simulink model "simTrabalho_CDU_sem_Desacoplador"  (R2018b)
settings: Solver=VariableStepAuto  StartTime=0.0  StopTime=tsim  MaxStep=1/10  RelTol=1e-3  EnableMultiTasking=on
values from neighbouring files (symbols this model uses):
  D = minreal(D)    [main.m]
  Dn = D    [main.m]
  G = G(iy,iu)    [main.m]
  u0 = u0(iu)    [main.m]
  umax = umax(iu)    [main.m]
  umin = umin(iu)    [main.m]
  y0 = y0(iy)    [main.m]
  ymax = ymax(iy)    [main.m]
  ymin = ymin(iy)    [main.m]
undefined symbols (not defined in the file or in its folder): Tdio
libraries: cstextras x36
settings Model: Creator=treezao  LastModifiedBy=Aluno
settings OptimizationCC: LifeSpan=inf
settings DebuggingCC: LibraryContextMissingDiagnostic=none  SFUnexpectedBacktrackingDiag=warning  SFNoUnconditionalDefaultTransitionDiag=warning  SFExecutionAtInitializationDiag=none
settings SFSimCC: SimUseLocalCustomCode=off
settings RTWCC: RTWUseLocalCustomCode=off
settings CodeAppCC: StateflowObjectComments=on
settings GRTTargetCC: TargetLangStandard=C89/C90 (ANSI)  GeneratePreprocessorConditionals=Disable all
settings ConfigComp: CovMetricSettings=dw  CovHtmlReporting=on  CovSaveCumulativeToWorkspaceVar=on  CovSaveSingleToWorkspaceVar=on  CovExternalEMLEnable=off

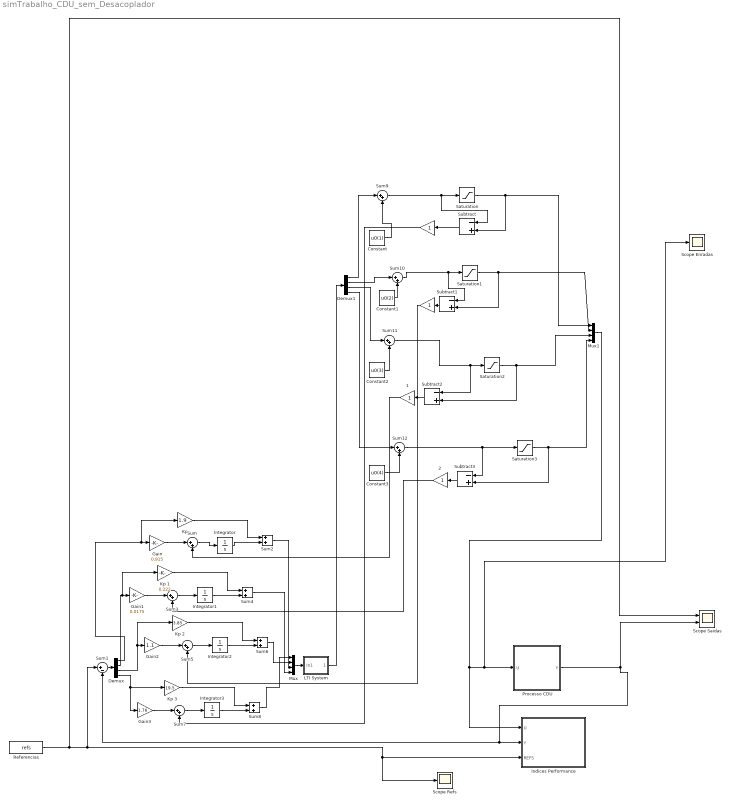
== system simTrabalho_CDU_sem_Desacoplador ==
   {,,1..2} (4 alike) : Gain
  Constant : Constant  Value=u0(1)
  Constant1 : Constant  Value=u0(2)
  Constant2 : Constant  Value=u0(3)
  Constant3 : Constant  Value=u0(4)
  Demux : Demux
  Demux1 : Demux
  Gain : Gain  Gain=0.915
  Gain1 : Gain  Gain=0.0175
  Gain2 : Gain  Gain=1.1
  Gain3 : Gain  Gain=1.76
  Indices Performance : Subsystem
  Integrator{,1..3} (4 alike) : Integrator
  "Kp " : Gain  Gain=1.9
  Kp 1 : Gain  Gain=0.222
  Kp 2 : Gain  Gain=3.85
  Kp 3 : Gain  Gain=19.5
  LTI System : Subsystem  AncestorBlock=cstblocks/LTI System  BlockChoice=CSS  mask(LTI Block){sys=Dn, IC=[]}
      mask prompts: sys "Control:simulink:LTIMaskLabel1"; IC "Control:simulink:LTIMaskLabel2"
      mask help: Control:simulink:LTIMaskDescription
      mask init:
      | try
      |    % read data to initialize mask variables
      |    [D,Ts,Tdi,Tdo,Tdio,x0,sysname]=...
      |       ltimask('Initialize',gcb,sys,IC);
      |    % update contents
      |    model = bdroot;
      |    df = get_param(model,'dirty');
      |    ltimask('UpdateDiagram',gcb,D,Ts,Tdio);
      |    try      
      |       % Attempt to modify locked library -> error
      |       % Makes block show ??? when loading CSTBLOCKS
      |       % for the first time
      |       set_param(model,'dirty',df)
      |    end
      | catch ME
      |    sys = [];  IC = [];   sysname = '???';
      |    throw(ME)
      | end
      mask Help: eval('ctrlguihelp(''ltisystemblock'');')
      mask Callback sys: ltimask('MaskLTICallback',gcb);
      mask Display: disp(sysname)
  Mux : Mux
  Mux1 : Mux
  Processo CDU : Subsystem
  Referencias : FromWorkspace  VariableName=refs  SampleTime=0  Interpolate=off  OutputAfterFinalValue=Holding final value
  Saturation : Saturate  UpperLimit=umax(1)  LowerLimit=umin(1)  LinearizeAsGain=off
  Saturation1 : Saturate  UpperLimit=umax(2)  LowerLimit=umin(2)  LinearizeAsGain=off
  Saturation2 : Saturate  UpperLimit=umax(3)  LowerLimit=umin(3)  LinearizeAsGain=off
  Saturation3 : Saturate  UpperLimit=umax(4)  LowerLimit=umin(4)  LinearizeAsGain=off
  Scope Enradas : Scope
  Scope Refs : Scope
  Scope Saidas : Scope  NumInputPorts=2
  Subtract{,1..3} (4 alike) : Sum  Inputs=-+
  Sum{,3,5,7,9..12} (8 alike) : Sum  Inputs=|++
  Sum1 : Sum  Inputs=|+-
  Sum{2,4,6,8} (4 alike) : Sum
  wires:
  Referencias/1 -> Scope Refs/1, Indices Performance/3(REFS), Sum1/1, Scope Saidas/1
  Demux/1 -> "Kp "/1, Gain/1
  Demux/2 -> Kp 1/1, Gain1/1
  Demux/3 -> Kp 2/1, Gain2/1
  Demux/4 -> Gain3/1, Kp 3/1
  Sum2/1 -> Mux/3
  Sum4/1 -> Mux/4
  Sum8/1 -> Mux/1
  Processo CDU/1(Y) -> Indices Performance/2(Y), Sum1/2, Scope Saidas/2
  Sum1/1 -> Demux/1
  Mux/1 -> LTI System/1(In1)
  Sum/1 -> Integrator/1
  Integrator/1 -> Sum2/2
  Gain/1 -> Sum/1
  "Kp "/1 -> Sum2/1
  Sum3/1 -> Integrator1/1
  Integrator1/1 -> Sum4/2
  Gain1/1 -> Sum3/1
  Kp 1/1 -> Sum4/1
  Sum5/1 -> Integrator2/1
  Integrator2/1 -> Sum6/2
  Gain2/1 -> Sum5/1
  Kp 2/1 -> Sum6/1
  Sum6/1 -> Mux/2
  Sum7/1 -> Integrator3/1
  Integrator3/1 -> Sum8/2
  Gain3/1 -> Sum7/1
  Kp 3/1 -> Sum8/1
  Subtract/1 -> " "/1
  Saturation/1 -> Subtract/2, Mux1/1
  Subtract1/1 -> " "/1
  Subtract2/1 -> " 1"/1
  Saturation1/1 -> Subtract1/2, Mux1/2
  Saturation2/1 -> Subtract2/2, Mux1/3
  Subtract3/1 -> " 2"/1
  Saturation3/1 -> Subtract3/2, Mux1/4
  Mux1/1 -> Indices Performance/1(U), Processo CDU/1(U), Scope Enradas/1
  LTI System/1(Out1) -> Demux1/1
  Sum9/1 -> Subtract/1, Saturation/1
  Demux1/1 -> Sum9/1
  Demux1/2 -> Sum10/1
  Sum10/1 -> Subtract1/1, Saturation1/1
  Demux1/3 -> Sum11/1
  Sum11/1 -> Subtract2/1, Saturation2/1
  Demux1/4 -> Sum12/1
  Sum12/1 -> Subtract3/1, Saturation3/1
  Constant/1 -> Sum9/2
  Constant1/1 -> Sum10/2
  Constant2/1 -> Sum11/2
  Constant3/1 -> Sum12/2
  " "/1 -> Sum5/2
  " "/1 -> Sum7/2
  " 1"/1 -> Sum/2
  " 2"/1 -> Sum3/2

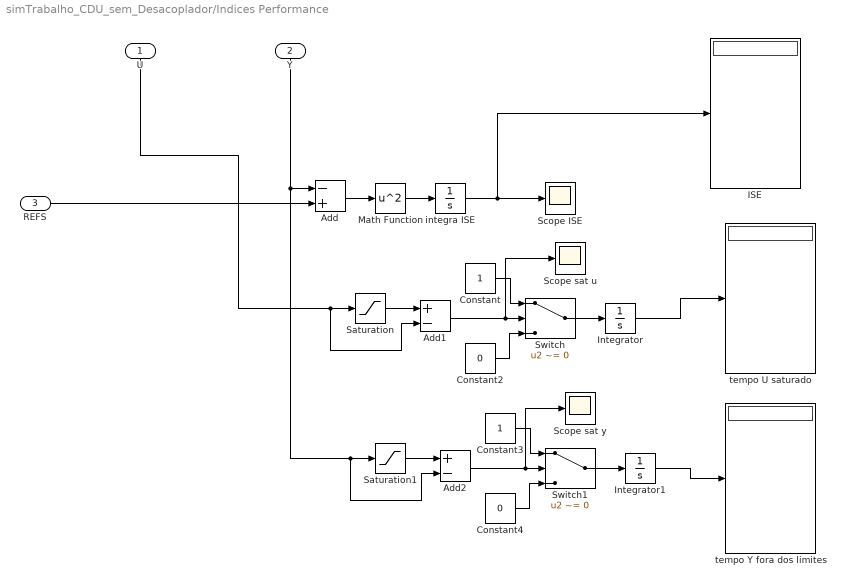
== system simTrabalho_CDU_sem_Desacoplador/Indices Performance ==
  U : Inport
  Y : Inport  Port=2
  REFS : Inport  Port=3
  Add : Sum  Inputs=-+
  Add1 : Sum  Inputs=+-
  Add2 : Sum  Inputs=+-
  Constant : Constant
  Constant2 : Constant  Value=0
  Constant3 : Constant
  Constant4 : Constant  Value=0
  ISE : Display
  Integrator : Integrator
  Integrator1 : Integrator
  Math Function : Math  Operator=square  SaturateOnIntegerOverflow=on
  Saturation : Saturate  UpperLimit=umax  LowerLimit=umin
  Saturation1 : Saturate  UpperLimit=ymax  LowerLimit=ymin
  Scope ISE : Scope
  Scope sat u : Scope
  Scope sat y : Scope
  Switch : Switch  Criteria=u2 ~= 0
  Switch1 : Switch  Criteria=u2 ~= 0
  integra ISE : Integrator
  tempo U saturado : Display
  tempo Y fora dos limites : Display
  wires:
  REFS/1 -> Add/2
  Y/1 -> Add2/2, Saturation1/1, Add/1
  U/1 -> Add1/2, Saturation/1
  Add2/1 -> Scope sat y/1, Switch1/2
  Constant3/1 -> Switch1/1
  Integrator1/1 -> tempo Y fora dos limites/1
  Constant4/1 -> Switch1/3
  Switch1/1 -> Integrator1/1
  Saturation1/1 -> Add2/1
  Saturation/1 -> Add1/1
  Constant2/1 -> Switch/3
  integra ISE/1 -> ISE/1, Scope ISE/1
  Constant/1 -> Switch/1
  Integrator/1 -> tempo U saturado/1
  Switch/1 -> Integrator/1
  Add1/1 -> Switch/2, Scope sat u/1
  Math Function/1 -> integra ISE/1
  Add/1 -> Math Function/1

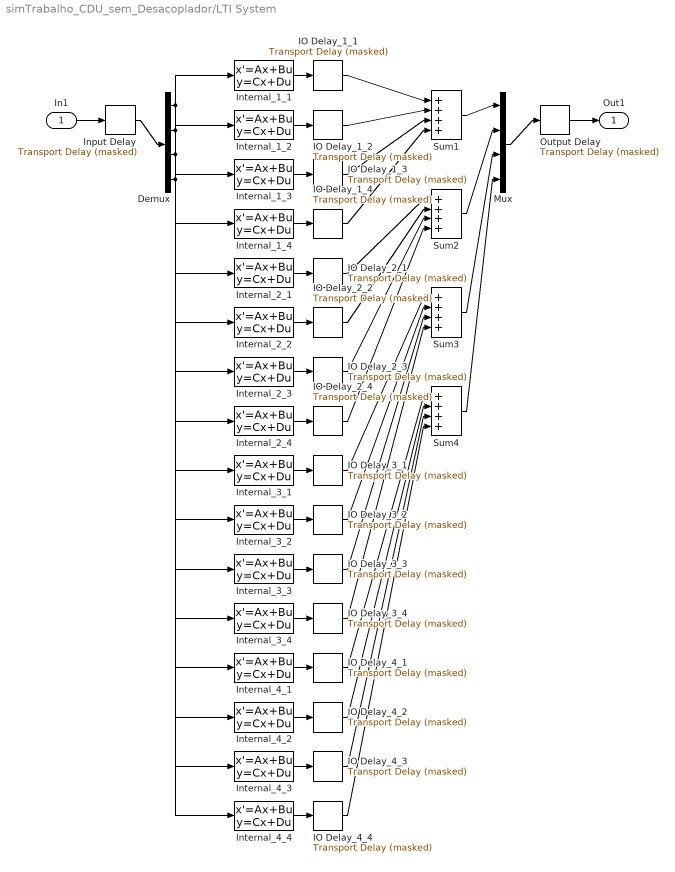
== system simTrabalho_CDU_sem_Desacoplador/LTI System ==
  In1 : Inport
  Demux : Demux
  IO Delay_1_1 : cstextras/Transport Delay (masked)  Td=Tdio(1,1)  u0=0  bufsize=1024
      settings: SourceProductName=Control System Toolbox  SourceProductBaseCode=CT
  IO Delay_1_2 : cstextras/Transport Delay (masked)  Td=Tdio(1,2)  u0=0  bufsize=1024
      settings: SourceProductName=Control System Toolbox  SourceProductBaseCode=CT
  IO Delay_1_3 : cstextras/Transport Delay (masked)  Td=Tdio(1,3)  u0=0  bufsize=1024
      settings: SourceProductName=Control System Toolbox  SourceProductBaseCode=CT
  IO Delay_1_4 : cstextras/Transport Delay (masked)  Td=Tdio(1,4)  u0=0  bufsize=1024
      settings: SourceProductName=Control System Toolbox  SourceProductBaseCode=CT
  IO Delay_2_1 : cstextras/Transport Delay (masked)  Td=Tdio(2,1)  u0=0  bufsize=1024
      settings: SourceProductName=Control System Toolbox  SourceProductBaseCode=CT
  IO Delay_2_2 : cstextras/Transport Delay (masked)  Td=Tdio(2,2)  u0=0  bufsize=1024
      settings: SourceProductName=Control System Toolbox  SourceProductBaseCode=CT
  IO Delay_2_3 : cstextras/Transport Delay (masked)  Td=Tdio(2,3)  u0=0  bufsize=1024
      settings: SourceProductName=Control System Toolbox  SourceProductBaseCode=CT
  IO Delay_2_4 : cstextras/Transport Delay (masked)  Td=Tdio(2,4)  u0=0  bufsize=1024
      settings: SourceProductName=Control System Toolbox  SourceProductBaseCode=CT
  IO Delay_3_1 : cstextras/Transport Delay (masked)  Td=Tdio(3,1)  u0=0  bufsize=1024
      settings: SourceProductName=Control System Toolbox  SourceProductBaseCode=CT
  IO Delay_3_2 : cstextras/Transport Delay (masked)  Td=Tdio(3,2)  u0=0  bufsize=1024
      settings: SourceProductName=Control System Toolbox  SourceProductBaseCode=CT
  IO Delay_3_3 : cstextras/Transport Delay (masked)  Td=Tdio(3,3)  u0=0  bufsize=1024
      settings: SourceProductName=Control System Toolbox  SourceProductBaseCode=CT
  IO Delay_3_4 : cstextras/Transport Delay (masked)  Td=Tdio(3,4)  u0=0  bufsize=1024
      settings: SourceProductName=Control System Toolbox  SourceProductBaseCode=CT
  IO Delay_4_1 : cstextras/Transport Delay (masked)  Td=Tdio(4,1)  u0=0  bufsize=1024
      settings: SourceProductName=Control System Toolbox  SourceProductBaseCode=CT
  IO Delay_4_2 : cstextras/Transport Delay (masked)  Td=Tdio(4,2)  u0=0  bufsize=1024
      settings: SourceProductName=Control System Toolbox  SourceProductBaseCode=CT
  IO Delay_4_3 : cstextras/Transport Delay (masked)  Td=Tdio(4,3)  u0=0  bufsize=1024
      settings: SourceProductName=Control System Toolbox  SourceProductBaseCode=CT
  IO Delay_4_4 : cstextras/Transport Delay (masked)  Td=Tdio(4,4)  u0=0  bufsize=1024
      settings: SourceProductName=Control System Toolbox  SourceProductBaseCode=CT
  Input Delay : cstextras/Transport Delay (masked)  Td=Tdi  u0=0  bufsize=1024
      settings: SourceProductName=Control System Toolbox  SourceProductBaseCode=CT
  Internal_1_1 : StateSpace  A=D(1,1).a  B=D(1,1).b  C=D(1,1).c  D=D(1,1).d
  Internal_1_2 : StateSpace  A=D(1,2).a  B=D(1,2).b  C=D(1,2).c  D=D(1,2).d
  Internal_1_3 : StateSpace  A=D(1,3).a  B=D(1,3).b  C=D(1,3).c  D=D(1,3).d
  Internal_1_4 : StateSpace  A=D(1,4).a  B=D(1,4).b  C=D(1,4).c  D=D(1,4).d
  Internal_2_1 : StateSpace  A=D(2,1).a  B=D(2,1).b  C=D(2,1).c  D=D(2,1).d
  Internal_2_2 : StateSpace  A=D(2,2).a  B=D(2,2).b  C=D(2,2).c  D=D(2,2).d
  Internal_2_3 : StateSpace  A=D(2,3).a  B=D(2,3).b  C=D(2,3).c  D=D(2,3).d
  Internal_2_4 : StateSpace  A=D(2,4).a  B=D(2,4).b  C=D(2,4).c  D=D(2,4).d
  Internal_3_1 : StateSpace  A=D(3,1).a  B=D(3,1).b  C=D(3,1).c  D=D(3,1).d
  Internal_3_2 : StateSpace  A=D(3,2).a  B=D(3,2).b  C=D(3,2).c  D=D(3,2).d
  Internal_3_3 : StateSpace  A=D(3,3).a  B=D(3,3).b  C=D(3,3).c  D=D(3,3).d
  Internal_3_4 : StateSpace  A=D(3,4).a  B=D(3,4).b  C=D(3,4).c  D=D(3,4).d
  Internal_4_1 : StateSpace  A=D(4,1).a  B=D(4,1).b  C=D(4,1).c  D=D(4,1).d
  Internal_4_2 : StateSpace  A=D(4,2).a  B=D(4,2).b  C=D(4,2).c  D=D(4,2).d
  Internal_4_3 : StateSpace  A=D(4,3).a  B=D(4,3).b  C=D(4,3).c  D=D(4,3).d
  Internal_4_4 : StateSpace  A=D(4,4).a  B=D(4,4).b  C=D(4,4).c  D=D(4,4).d
  Mux : Mux
  Output Delay : cstextras/Transport Delay (masked)  Td=Tdo  u0=0  bufsize=1024
      settings: SourceProductName=Control System Toolbox  SourceProductBaseCode=CT
  Sum{1..4} (4 alike) : Sum  Inputs=++++  SaturateOnIntegerOverflow=on  InputSameDT=on  OutDataTypeStr=Inherit: Same as first input
  Out1 : Outport  InitialOutput=0
  wires:
  In1/1 -> Input Delay/1
  Output Delay/1 -> Out1/1
  Input Delay/1 -> Demux/1
  Mux/1 -> Output Delay/1
  Sum1/1 -> Mux/1
  Sum2/1 -> Mux/2
  Sum3/1 -> Mux/3
  Sum4/1 -> Mux/4
  Demux/1 -> Internal_1_1/1, Internal_2_1/1, Internal_3_1/1, Internal_4_1/1
  Internal_1_1/1 -> IO Delay_1_1/1
  IO Delay_1_1/1 -> Sum1/1
  Demux/2 -> Internal_1_2/1, Internal_2_2/1, Internal_3_2/1, Internal_4_2/1
  Internal_1_2/1 -> IO Delay_1_2/1
  IO Delay_1_2/1 -> Sum1/2
  Demux/3 -> Internal_1_3/1, Internal_2_3/1, Internal_3_3/1, Internal_4_3/1
  Internal_1_3/1 -> IO Delay_1_3/1
  IO Delay_1_3/1 -> Sum1/3
  Demux/4 -> Internal_1_4/1, Internal_2_4/1, Internal_3_4/1, Internal_4_4/1
  Internal_1_4/1 -> IO Delay_1_4/1
  IO Delay_1_4/1 -> Sum1/4
  Internal_2_1/1 -> IO Delay_2_1/1
  IO Delay_2_1/1 -> Sum2/1
  Internal_2_2/1 -> IO Delay_2_2/1
  IO Delay_2_2/1 -> Sum2/2
  Internal_2_3/1 -> IO Delay_2_3/1
  IO Delay_2_3/1 -> Sum2/3
  Internal_2_4/1 -> IO Delay_2_4/1
  IO Delay_2_4/1 -> Sum2/4
  Internal_3_1/1 -> IO Delay_3_1/1
  IO Delay_3_1/1 -> Sum3/1
  Internal_3_2/1 -> IO Delay_3_2/1
  IO Delay_3_2/1 -> Sum3/2
  Internal_3_3/1 -> IO Delay_3_3/1
  IO Delay_3_3/1 -> Sum3/3
  Internal_3_4/1 -> IO Delay_3_4/1
  IO Delay_3_4/1 -> Sum3/4
  Internal_4_1/1 -> IO Delay_4_1/1
  IO Delay_4_1/1 -> Sum4/1
  Internal_4_2/1 -> IO Delay_4_2/1
  IO Delay_4_2/1 -> Sum4/2
  Internal_4_3/1 -> IO Delay_4_3/1
  IO Delay_4_3/1 -> Sum4/3
  Internal_4_4/1 -> IO Delay_4_4/1
  IO Delay_4_4/1 -> Sum4/4

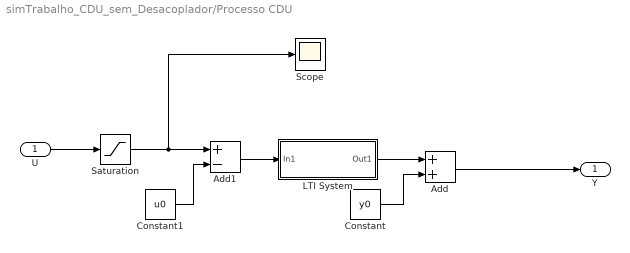
== system simTrabalho_CDU_sem_Desacoplador/Processo CDU ==
  U : Inport
  Add : Sum
  Add1 : Sum  Inputs=+-
  Constant : Constant  Value=y0
  Constant1 : Constant  Value=u0
  LTI System : Subsystem  AncestorBlock=cstblocks/LTI System  BlockChoice=CSS  mask(LTI Block){sys=G, IC=[]}
      mask prompts: sys "Control:simulink:LTIMaskLabel1"; IC "Control:simulink:LTIMaskLabel2"
      mask help: Control:simulink:LTIMaskDescription
      mask init: same as simTrabalho_CDU_sem_Desacoplador/LTI System
      mask Help: eval('ctrlguihelp(''ltisystemblock'');')
      mask Callback sys: ltimask('MaskLTICallback',gcb);
      mask Display: disp(sysname)
  Saturation : Saturate  UpperLimit=umax  LowerLimit=umin
  Scope : Scope
  Y : Outport
  wires:
  LTI System/1(Out1) -> Add/1
  U/1 -> Saturation/1
  Add1/1 -> LTI System/1(In1)
  Constant/1 -> Add/2
  Add/1 -> Y/1
  Constant1/1 -> Add1/2
  Saturation/1 -> Scope/1, Add1/1

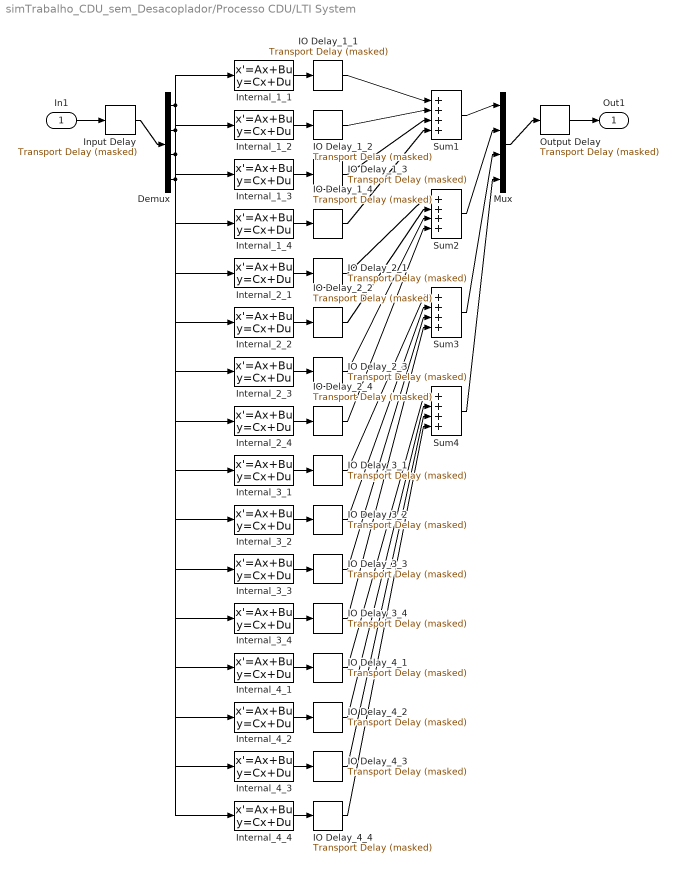
== system simTrabalho_CDU_sem_Desacoplador/Processo CDU/LTI System ==
  In1 : Inport
  Demux : Demux
  IO Delay_1_1 : cstextras/Transport Delay (masked)  Td=Tdio(1,1)  u0=0  bufsize=1024
      settings: SourceProductName=Control System Toolbox  SourceProductBaseCode=CT
  IO Delay_1_2 : cstextras/Transport Delay (masked)  Td=Tdio(1,2)  u0=0  bufsize=1024
      settings: SourceProductName=Control System Toolbox  SourceProductBaseCode=CT
  IO Delay_1_3 : cstextras/Transport Delay (masked)  Td=Tdio(1,3)  u0=0  bufsize=1024
      settings: SourceProductName=Control System Toolbox  SourceProductBaseCode=CT
  IO Delay_1_4 : cstextras/Transport Delay (masked)  Td=Tdio(1,4)  u0=0  bufsize=1024
      settings: SourceProductName=Control System Toolbox  SourceProductBaseCode=CT
  IO Delay_2_1 : cstextras/Transport Delay (masked)  Td=Tdio(2,1)  u0=0  bufsize=1024
      settings: SourceProductName=Control System Toolbox  SourceProductBaseCode=CT
  IO Delay_2_2 : cstextras/Transport Delay (masked)  Td=Tdio(2,2)  u0=0  bufsize=1024
      settings: SourceProductName=Control System Toolbox  SourceProductBaseCode=CT
  IO Delay_2_3 : cstextras/Transport Delay (masked)  Td=Tdio(2,3)  u0=0  bufsize=1024
      settings: SourceProductName=Control System Toolbox  SourceProductBaseCode=CT
  IO Delay_2_4 : cstextras/Transport Delay (masked)  Td=Tdio(2,4)  u0=0  bufsize=1024
      settings: SourceProductName=Control System Toolbox  SourceProductBaseCode=CT
  IO Delay_3_1 : cstextras/Transport Delay (masked)  Td=Tdio(3,1)  u0=0  bufsize=1024
      settings: SourceProductName=Control System Toolbox  SourceProductBaseCode=CT
  IO Delay_3_2 : cstextras/Transport Delay (masked)  Td=Tdio(3,2)  u0=0  bufsize=1024
      settings: SourceProductName=Control System Toolbox  SourceProductBaseCode=CT
  IO Delay_3_3 : cstextras/Transport Delay (masked)  Td=Tdio(3,3)  u0=0  bufsize=1024
      settings: SourceProductName=Control System Toolbox  SourceProductBaseCode=CT
  IO Delay_3_4 : cstextras/Transport Delay (masked)  Td=Tdio(3,4)  u0=0  bufsize=1024
      settings: SourceProductName=Control System Toolbox  SourceProductBaseCode=CT
  IO Delay_4_1 : cstextras/Transport Delay (masked)  Td=Tdio(4,1)  u0=0  bufsize=1024
      settings: SourceProductName=Control System Toolbox  SourceProductBaseCode=CT
  IO Delay_4_2 : cstextras/Transport Delay (masked)  Td=Tdio(4,2)  u0=0  bufsize=1024
      settings: SourceProductName=Control System Toolbox  SourceProductBaseCode=CT
  IO Delay_4_3 : cstextras/Transport Delay (masked)  Td=Tdio(4,3)  u0=0  bufsize=1024
      settings: SourceProductName=Control System Toolbox  SourceProductBaseCode=CT
  IO Delay_4_4 : cstextras/Transport Delay (masked)  Td=Tdio(4,4)  u0=0  bufsize=1024
      settings: SourceProductName=Control System Toolbox  SourceProductBaseCode=CT
  Input Delay : cstextras/Transport Delay (masked)  Td=Tdi  u0=0  bufsize=1024
      settings: SourceProductName=Control System Toolbox  SourceProductBaseCode=CT
  Internal_1_1 : StateSpace  A=D(1,1).a  B=D(1,1).b  C=D(1,1).c  D=D(1,1).d
  Internal_1_2 : StateSpace  A=D(1,2).a  B=D(1,2).b  C=D(1,2).c  D=D(1,2).d
  Internal_1_3 : StateSpace  A=D(1,3).a  B=D(1,3).b  C=D(1,3).c  D=D(1,3).d
  Internal_1_4 : StateSpace  A=D(1,4).a  B=D(1,4).b  C=D(1,4).c  D=D(1,4).d
  Internal_2_1 : StateSpace  A=D(2,1).a  B=D(2,1).b  C=D(2,1).c  D=D(2,1).d
  Internal_2_2 : StateSpace  A=D(2,2).a  B=D(2,2).b  C=D(2,2).c  D=D(2,2).d
  Internal_2_3 : StateSpace  A=D(2,3).a  B=D(2,3).b  C=D(2,3).c  D=D(2,3).d
  Internal_2_4 : StateSpace  A=D(2,4).a  B=D(2,4).b  C=D(2,4).c  D=D(2,4).d
  Internal_3_1 : StateSpace  A=D(3,1).a  B=D(3,1).b  C=D(3,1).c  D=D(3,1).d
  Internal_3_2 : StateSpace  A=D(3,2).a  B=D(3,2).b  C=D(3,2).c  D=D(3,2).d
  Internal_3_3 : StateSpace  A=D(3,3).a  B=D(3,3).b  C=D(3,3).c  D=D(3,3).d
  Internal_3_4 : StateSpace  A=D(3,4).a  B=D(3,4).b  C=D(3,4).c  D=D(3,4).d
  Internal_4_1 : StateSpace  A=D(4,1).a  B=D(4,1).b  C=D(4,1).c  D=D(4,1).d
  Internal_4_2 : StateSpace  A=D(4,2).a  B=D(4,2).b  C=D(4,2).c  D=D(4,2).d
  Internal_4_3 : StateSpace  A=D(4,3).a  B=D(4,3).b  C=D(4,3).c  D=D(4,3).d
  Internal_4_4 : StateSpace  A=D(4,4).a  B=D(4,4).b  C=D(4,4).c  D=D(4,4).d
  Mux : Mux
  Output Delay : cstextras/Transport Delay (masked)  Td=Tdo  u0=0  bufsize=1024
      settings: SourceProductName=Control System Toolbox  SourceProductBaseCode=CT
  Sum{1..4} (4 alike) : Sum  Inputs=++++  SaturateOnIntegerOverflow=on  InputSameDT=on  OutDataTypeStr=Inherit: Same as first input
  Out1 : Outport  InitialOutput=0
  wires:
  In1/1 -> Input Delay/1
  Output Delay/1 -> Out1/1
  Input Delay/1 -> Demux/1
  Mux/1 -> Output Delay/1
  Sum1/1 -> Mux/1
  Sum2/1 -> Mux/2
  Sum3/1 -> Mux/3
  Sum4/1 -> Mux/4
  Demux/1 -> Internal_1_1/1, Internal_2_1/1, Internal_3_1/1, Internal_4_1/1
  Internal_1_1/1 -> IO Delay_1_1/1
  IO Delay_1_1/1 -> Sum1/1
  Demux/2 -> Internal_1_2/1, Internal_2_2/1, Internal_3_2/1, Internal_4_2/1
  Internal_1_2/1 -> IO Delay_1_2/1
  IO Delay_1_2/1 -> Sum1/2
  Demux/3 -> Internal_1_3/1, Internal_2_3/1, Internal_3_3/1, Internal_4_3/1
  Internal_1_3/1 -> IO Delay_1_3/1
  IO Delay_1_3/1 -> Sum1/3
  Demux/4 -> Internal_1_4/1, Internal_2_4/1, Internal_3_4/1, Internal_4_4/1
  Internal_1_4/1 -> IO Delay_1_4/1
  IO Delay_1_4/1 -> Sum1/4
  Internal_2_1/1 -> IO Delay_2_1/1
  IO Delay_2_1/1 -> Sum2/1
  Internal_2_2/1 -> IO Delay_2_2/1
  IO Delay_2_2/1 -> Sum2/2
  Internal_2_3/1 -> IO Delay_2_3/1
  IO Delay_2_3/1 -> Sum2/3
  Internal_2_4/1 -> IO Delay_2_4/1
  IO Delay_2_4/1 -> Sum2/4
  Internal_3_1/1 -> IO Delay_3_1/1
  IO Delay_3_1/1 -> Sum3/1
  Internal_3_2/1 -> IO Delay_3_2/1
  IO Delay_3_2/1 -> Sum3/2
  Internal_3_3/1 -> IO Delay_3_3/1
  IO Delay_3_3/1 -> Sum3/3
  Internal_3_4/1 -> IO Delay_3_4/1
  IO Delay_3_4/1 -> Sum3/4
  Internal_4_1/1 -> IO Delay_4_1/1
  IO Delay_4_1/1 -> Sum4/1
  Internal_4_2/1 -> IO Delay_4_2/1
  IO Delay_4_2/1 -> Sum4/2
  Internal_4_3/1 -> IO Delay_4_3/1
  IO Delay_4_3/1 -> Sum4/3
  Internal_4_4/1 -> IO Delay_4_4/1
  IO Delay_4_4/1 -> Sum4/4
